simulink library "AERO"  (R2016b)
settings: Solver=VariableStepAuto  StartTime=0.0  StopTime=10.0  RelTol=1e-3
values from neighbouring files (symbols this model uses):
  AERO = AEROmod    [setup_aero.m]
libraries: FIN x4
settings Model: Creator=Andrew  LastModifiedBy=Andrew

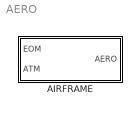
== system AERO ==
  AIRFRAME : Subsystem

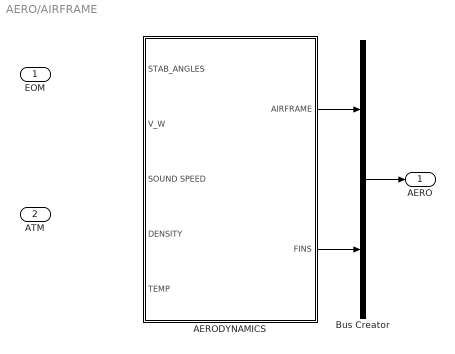
== system AERO/AIRFRAME ==
  EOM : Inport
  ATM : Inport  Port=2
  AERODYNAMICS : Subsystem
  Bus Creator : BusCreator  Inputs=2
  AERO : Outport
  wires:
  AERODYNAMICS/1(AIRFRAME) -> Bus Creator/1
  AERODYNAMICS/2(FINS) -> Bus Creator/2
  Bus Creator/1 -> AERO/1

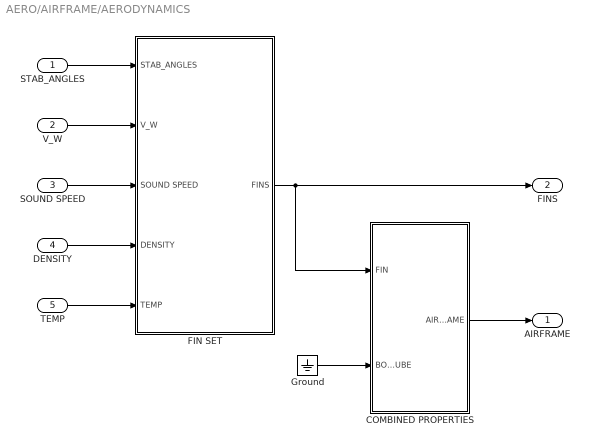
== system AERO/AIRFRAME/AERODYNAMICS ==
  STAB_ANGLES : Inport
  V_W : Inport  Port=2
  SOUND SPEED : Inport  Port=3
  DENSITY : Inport  Port=4
  TEMP : Inport  Port=5
  COMBINED PROPERTIES : Subsystem
  FIN SET : Subsystem
  Ground : Ground
  AIRFRAME : Outport
  FINS : Outport  Port=2
  wires:
  V_W/1 -> FIN SET/2(V_W)
  SOUND SPEED/1 -> FIN SET/3(SOUND SPEED)
  STAB_ANGLES/1 -> FIN SET/1(STAB_ANGLES)
  DENSITY/1 -> FIN SET/4(DENSITY)
  TEMP/1 -> FIN SET/5(TEMP)
  FIN SET/1(FINS) -> COMBINED PROPERTIES/1(FIN), FINS/1
  COMBINED PROPERTIES/1(AIRFRAME) -> AIRFRAME/1
  Ground/1 -> COMBINED PROPERTIES/2(BODY_TUBE)

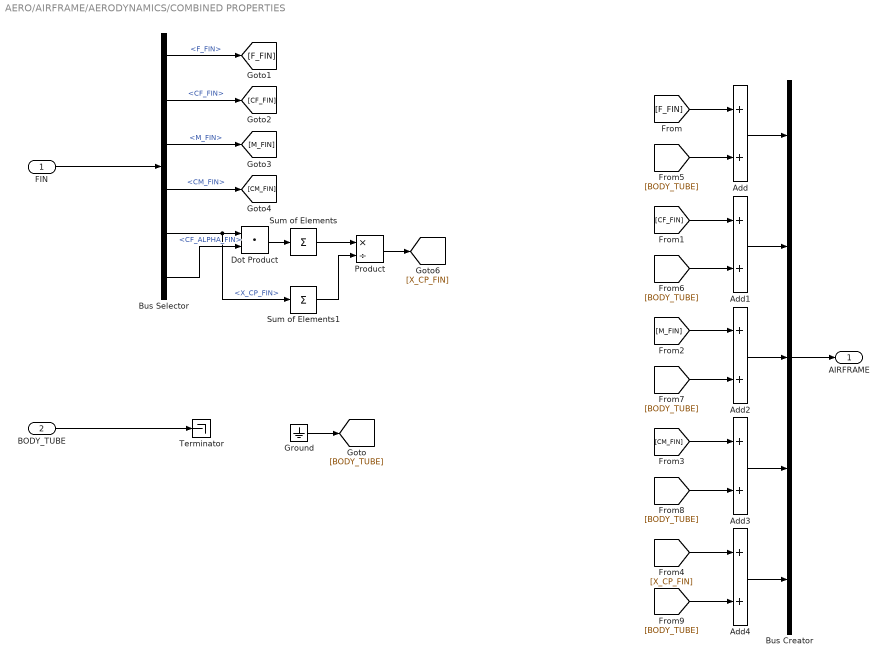
== system AERO/AIRFRAME/AERODYNAMICS/COMBINED PROPERTIES ==
  FIN : Inport
  BODY_TUBE : Inport  Port=2
  Add{,1..4} (5 alike) : Sum
  Bus Creator : BusCreator  Inputs=5
  Bus Selector : BusSelector  OutputSignals=F_FIN,CF_FIN,M_FIN,CM_FIN,X_CP_FIN,CF_ALPHA_FIN
  Dot Product : DotProduct  InputSameDT=on  OutDataTypeStr=Inherit: Inherit via internal rule
  Ground : Ground
  Product : Product  Inputs=*/
  Sum of Elements : Sum  Inputs=+
  Sum of Elements1 : Sum  Inputs=+
  Terminator : Terminator
  AIRFRAME : Outport
  wires:
  Bus Selector/5 -> Sum of Elements1/1, Dot Product/1  "<X_CP_FIN>"
  Dot Product/1 -> Sum of Elements/1
  Bus Selector/6 -> Dot Product/2  "<CF_ALPHA_FIN>"
  Sum of Elements/1 -> Product/1
  Sum of Elements1/1 -> Product/2
  FIN/1 -> Bus Selector/1
  Bus Creator/1 -> AIRFRAME/1
  Add/1 -> Bus Creator/1
  Add1/1 -> Bus Creator/2
  Add2/1 -> Bus Creator/3
  Add4/1 -> Bus Creator/5
  Add3/1 -> Bus Creator/4
  BODY_TUBE/1 -> Terminator/1
  Ground/1 -> [BODY_TUBE]
  Bus Selector/1 -> [F_FIN]  "<F_FIN>"
  Bus Selector/2 -> [CF_FIN]  "<CF_FIN>"
  Bus Selector/3 -> [M_FIN]  "<M_FIN>"
  Bus Selector/4 -> [CM_FIN]  "<CM_FIN>"
  Product/1 -> [X_CP_FIN]
  [F_FIN] -> Add/1
  [CF_FIN] -> Add1/1
  [M_FIN] -> Add2/1
  [CM_FIN] -> Add3/1
  [X_CP_FIN] -> Add4/1
  [BODY_TUBE] -> Add/2
  [BODY_TUBE] -> Add1/2
  [BODY_TUBE] -> Add3/2
  [BODY_TUBE] -> Add4/2
  [BODY_TUBE] -> Add2/2

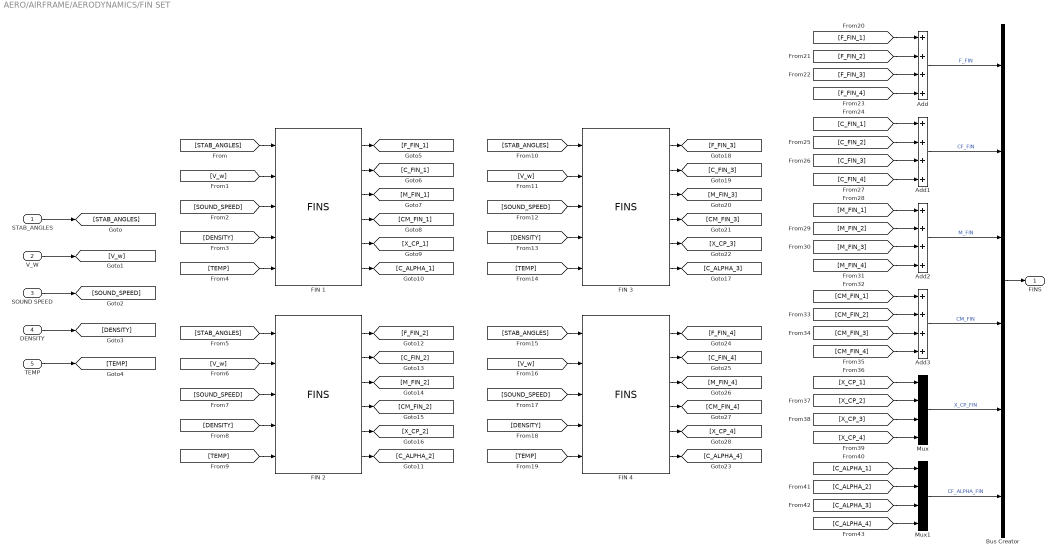
== system AERO/AIRFRAME/AERODYNAMICS/FIN SET ==
  STAB_ANGLES : Inport
  V_W : Inport  Port=2
  SOUND SPEED : Inport  Port=3
  DENSITY : Inport  Port=4
  TEMP : Inport  Port=5
  Add{,1..3} (4 alike) : Sum  Inputs=++++
  Bus Creator : BusCreator  Inputs=6
  FIN 1 : FIN/FINS  FIN=AERO.FIN(1)
  FIN 2 : FIN/FINS  FIN=AERO.FIN(2)
  FIN 3 : FIN/FINS  FIN=AERO.FIN(3)
  FIN 4 : FIN/FINS  FIN=AERO.FIN(4)
  Mux : Mux
  Mux1 : Mux
  FINS : Outport
  wires:
  STAB_ANGLES/1 -> [STAB_ANGLES]
  V_W/1 -> [V_w]
  SOUND SPEED/1 -> [SOUND_SPEED]
  DENSITY/1 -> [DENSITY]
  TEMP/1 -> [TEMP]
  [STAB_ANGLES] -> FIN 1/1
  [V_w] -> FIN 1/2
  [SOUND_SPEED] -> FIN 1/3
  [DENSITY] -> FIN 1/4
  [TEMP] -> FIN 1/5
  [DENSITY] -> FIN 2/4
  [STAB_ANGLES] -> FIN 2/1
  [V_w] -> FIN 2/2
  [SOUND_SPEED] -> FIN 2/3
  [TEMP] -> FIN 2/5
  [STAB_ANGLES] -> FIN 3/1
  [DENSITY] -> FIN 3/4
  [SOUND_SPEED] -> FIN 3/3
  [TEMP] -> FIN 3/5
  [V_w] -> FIN 3/2
  [STAB_ANGLES] -> FIN 4/1
  [V_w] -> FIN 4/2
  [DENSITY] -> FIN 4/4
  [SOUND_SPEED] -> FIN 4/3
  [TEMP] -> FIN 4/5
  FIN 1/1 -> [F_FIN_1]
  FIN 1/2 -> [C_FIN_1]
  FIN 1/3 -> [M_FIN_1]
  FIN 1/4 -> [CM_FIN_1]
  FIN 1/5 -> [X_CP_1]
  FIN 1/6 -> [C_ALPHA_1]
  FIN 2/1 -> [F_FIN_2]
  FIN 2/2 -> [C_FIN_2]
  FIN 2/3 -> [M_FIN_2]
  FIN 2/4 -> [CM_FIN_2]
  FIN 2/5 -> [X_CP_2]
  FIN 2/6 -> [C_ALPHA_2]
  FIN 3/1 -> [F_FIN_3]
  FIN 3/2 -> [C_FIN_3]
  FIN 3/3 -> [M_FIN_3]
  FIN 3/4 -> [CM_FIN_3]
  FIN 3/5 -> [X_CP_3]
  FIN 3/6 -> [C_ALPHA_3]
  FIN 4/1 -> [F_FIN_4]
  FIN 4/2 -> [C_FIN_4]
  FIN 4/3 -> [M_FIN_4]
  FIN 4/4 -> [CM_FIN_4]
  FIN 4/5 -> [X_CP_4]
  FIN 4/6 -> [C_ALPHA_4]
  [F_FIN_1] -> Add/1
  [F_FIN_2] -> Add/2
  [F_FIN_3] -> Add/3
  [F_FIN_4] -> Add/4
  Add/1 -> Bus Creator/1  "F_FIN"
  [C_FIN_1] -> Add1/1
  [C_FIN_2] -> Add1/2
  [C_FIN_3] -> Add1/3
  [C_FIN_4] -> Add1/4
  Add1/1 -> Bus Creator/2  "CF_FIN"
  [M_FIN_1] -> Add2/1
  [M_FIN_2] -> Add2/2
  [M_FIN_3] -> Add2/3
  [M_FIN_4] -> Add2/4
  Add2/1 -> Bus Creator/3  "M_FIN"
  [CM_FIN_1] -> Add3/1
  [CM_FIN_2] -> Add3/2
  [CM_FIN_3] -> Add3/3
  [CM_FIN_4] -> Add3/4
  Add3/1 -> Bus Creator/4  "CM_FIN"
  [X_CP_1] -> Mux/1
  [X_CP_2] -> Mux/2
  [X_CP_3] -> Mux/3
  [X_CP_4] -> Mux/4
  Mux/1 -> Bus Creator/5  "X_CP_FIN"
  [C_ALPHA_1] -> Mux1/1
  [C_ALPHA_2] -> Mux1/2
  [C_ALPHA_3] -> Mux1/3
  [C_ALPHA_4] -> Mux1/4
  Mux1/1 -> Bus Creator/6  "CF_ALPHA_FIN"
  Bus Creator/1 -> FINS/1
